simulink model "prac_p3"  (R2024a)
settings: Solver=VariableStepAuto  StartTime=0.0  StopTime=2200  RelTol=1e-3
libraries: simulink x2, slpidlib x1
settings Model: Creator=heman  LastModifiedBy=heman

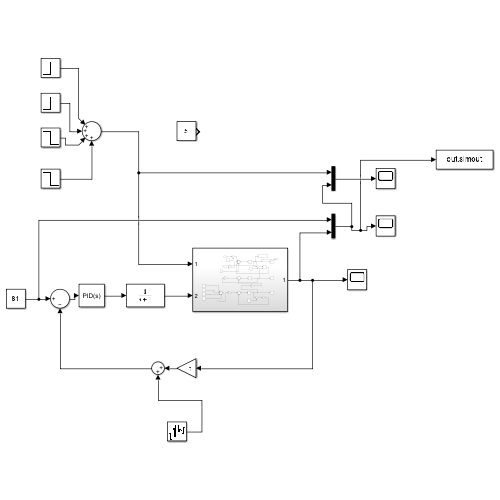
[thumbnail: Simulink's stored preview of the top-level diagram]
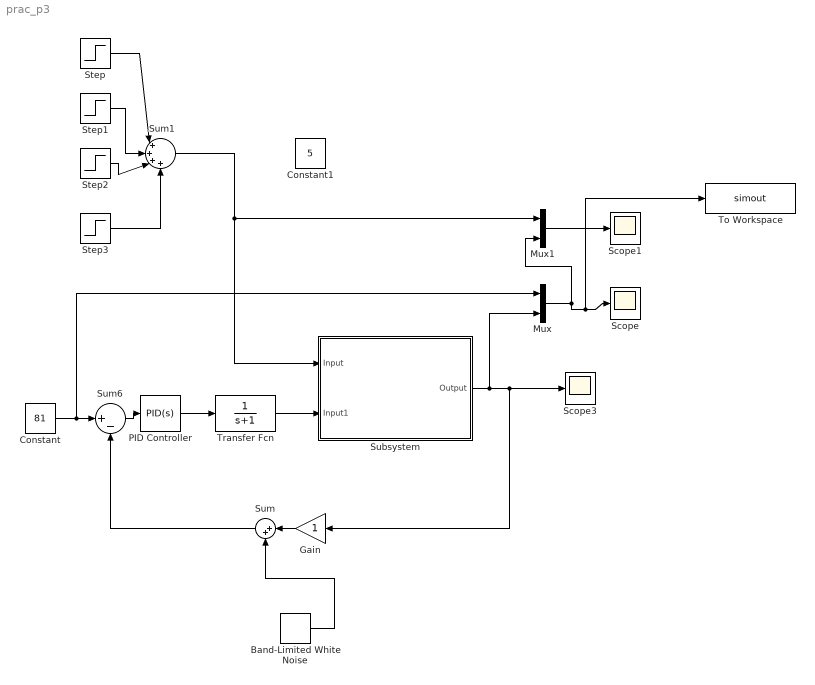
== system prac_p3 ==
  Band-Limited White Noise : simulink/Sources/Band-Limited White Noise  Cov=[0.1]  Ts=0.1  seed=[23341]
  Constant : Constant  Value=81
  Constant1 : Constant  Value=5
  Gain : Gain
  Mux : Mux  Inputs=2
  Mux1 : Mux  Inputs=2
  PID Controller : slpidlib/PID Controller  Controller=PID  Form=Ideal  TimeDomain=Continuous-time  UseExternalTs=off  SampleTime=-1  IntegratorMethod=Forward Euler  FilterMethod=Forward Euler  ControllerParametersSource=internal  P=-0.5078  I=0.01557  UseKiTs=off  D=15.92  UseExternalDerivativeSource=off  N=5.876  UseFilter=on  TunerSelectOption=Transfer Function Based (PID Tuner App)  InitialConditionSource=internal  InitialConditionForIntegrator=0  InitialConditionForFilter=0  DifferentiatorICPrevScaledInput=0  ExternalReset=none  TrackingMode=off  Kt=1  LimitOutput=off  SatLimitsSource=internal  UpperSaturationLimit=inf  LowerSaturationLimit=-inf  LinearizeAsGain=on  AntiWindupMode=none  Kb=1  LimitIntegrator=off  UpperIntegratorSaturationLimit=inf  LowerIntegratorSaturationLimit=-inf  POutMin=[]  POutMax=[]  IOutMin=[]  IOutMax=[]  DOutMin=[]  DOutMax=[]  NOutMin=[]  NOutMax=[]  SumOutMin=[]  SumOutMax=[]  SaturationOutMin=[]  SaturationOutMax=[]  PParamMin=[]  PParamMax=[]  IParamMin=[]  IParamMax=[]  DParamMin=[]  DParamMax=[]  NParamMin=[]  NParamMax=[]  KbParamMin=[]  KbParamMax=[]  KtParamMin=[]  KtParamMax=[]  KbOutMin=[]  KbOutMax=[]  KtOutMin=[]  KtOutMax=[]  IntegratorOutMin=[]  IntegratorOutMax=[]  FilterOutMin=[]  FilterOutMax=[]  SumI1OutMin=[]  SumI1OutMax=[]  SumI2OutMin=[]  SumI2OutMax=[]  SumI3OutMin=[]  SumI3OutMax=[]  SumI4OutMin=[]  SumI4OutMax=[]  SumDOutMin=[]  SumDOutMax=[]  DifferentiatorOutMin=[]  DifferentiatorOutMax=[]  FilterDiffOutCoefMin=[]  FilterDiffOutCoefMax=[]  ReciprocalOutMin=[]  ReciprocalOutMax=[]  SumDenOutMin=[]  SumDenOutMax=[]  SumNumOutMin=[]  SumNumOutMax=[]  DivideOutMin=[]  DivideOutMax=[]  UdiffTsProdOutMin=[]  UdiffTsProdOutMax=[]  NTsProdOutMin=[]  NTsProdOutMax=[]  UintegralTsProdOutMin=[]  UintegralTsProdOutMax=[]  UngainTsProdOutMin=[]  UngainTsProdOutMax=[]  ClampingZeroOutDataTypeStr=Inherit: Inherit via back propagation  ClampingZeroOutMin=[]  ClampingZeroOutMax=[]  FilterDenConstantOutDataTypeStr=Inherit: Inherit via back propagation  FilterDenConstantOutMin=[]  FilterDenConstantOutMax=[]  PCopyOutDataTypeStr=Inherit: Inherit via back propagation  PCopyOutMin=[]  PCopyOutMax=[]  NCopyOutDataTypeStr=Inherit: Inherit via back propagation  NCopyOutMin=[]  NCopyOutMax=[]  IntegratorContinuousStateAttributes=''  IntegratorStateMustResolveToSignalObject=off  IntegratorRTWStateStorageClass=Auto  FilterContinuousStateAttributes=''  FilterStateMustResolveToSignalObject=off  FilterRTWStateStorageClass=Auto  ParallelPVariant=Passthrough  IdealPVariant=InternalParameters  IVariant=InternalParameters  DVariant=InternalParameters  IntegratorVariant=Continuous  SatVariant=Disabled  AWVariant=Passthrough  PCopyVariant=Disabled  TRVariant=Disabled  FdbkBlocksVariant=Forward  IdealPFdbkVariant=Disabled  SatFdbkVariant=Disabled  DerivativeFilterVariant=ContFilter  NVariant=InternalParameters  NCopyVariant=Disabled  FilterICVariant=InternalICsFilter  IntegratorICVariant=InternalICs  ExternalResetVariant=Disabled  TRSumVariant=Passthrough  SumFdbkVariant=Disabled  SumVariant=Sum_PID  TsampFilterVariant=InternalTs  TsampNgainVariant=Passthrough  TsampIntegralVariant=Disabled_SignalSpec  ExternalSaturationOutDataTypeStr=Inherit: Same as second input  DerivativeSourceVariant=ErrorSignal
  Scope : Scope
  Scope1 : Scope
  Scope3 : Scope
  Step : Step  Time=400  Before=5  After=10  SampleTime=0
  Step1 : Step  Time=800  After=5  SampleTime=0
  Step2 : Step  Time=1200  After=-5  SampleTime=0
  Step3 : Step  Time=1600  After=-5  SampleTime=0
  Subsystem : Subsystem
  Sum : Sum  Inputs=|++
  Sum1 : Sum  Inputs=|++++
  Sum6 : Sum  Inputs=|+-
  To Workspace : ToWorkspace  VariableName=simout  SampleTime=-1
  Transfer Fcn : TransferFcn  Denominator=[1 1]
  wires:
  Transfer Fcn/1 -> Subsystem/2(Input1)
  Sum1/1 -> Mux1/1, Subsystem/1(Input)
  PID Controller/1 -> Transfer Fcn/1
  Subsystem/1(Output) -> Scope3/1, Gain/1, Mux/2
  Sum6/1 -> PID Controller/1
  Gain/1 -> Sum/1
  Band-Limited White Noise/1 -> Sum/2
  Sum/1 -> Sum6/2
  Constant/1 -> Mux/1, Sum6/1
  Mux/1 -> Mux1/2, To Workspace/1, Scope/1
  Step2/1 -> Sum1/3
  Step/1 -> Sum1/1
  Step3/1 -> Sum1/4
  Step1/1 -> Sum1/2
  Mux1/1 -> Scope1/1

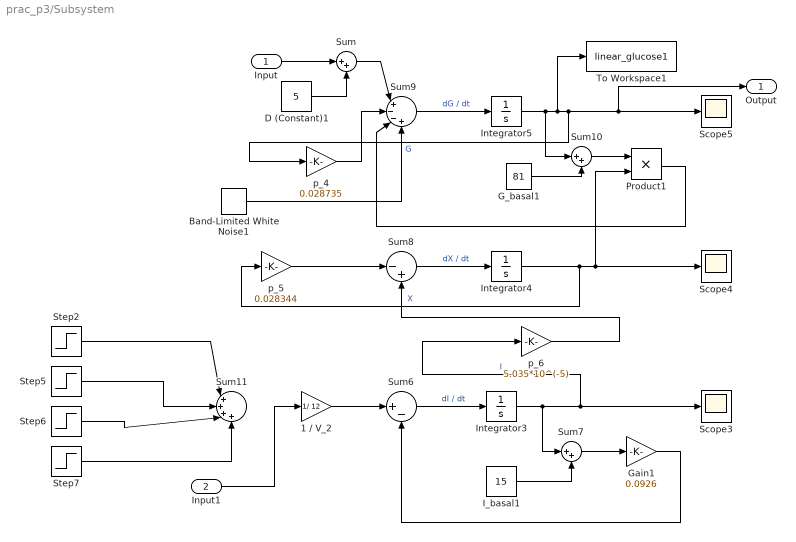
== system prac_p3/Subsystem ==
  Input : Inport
  Input1 : Inport  Port=2
  1 / V_2 : Gain  Gain=1/ 12
  Band-Limited White Noise1 : simulink/Sources/Band-Limited White Noise  Cov=[0.1]  Ts=0.1  seed=[23341]
  D (Constant)1 : Constant  Value=5
  G_basal1 : Constant  Value=81
  Gain1 : Gain  Gain=0.0926
  I_basal1 : Constant  Value=15
  Integrator3 : Integrator
  Integrator4 : Integrator
  Integrator5 : Integrator
  Product1 : Product
  Scope3 : Scope
  Scope4 : Scope
  Scope5 : Scope
  Step2 : Step  Time=500  Before=25  After=27.5  SampleTime=0
  Step5 : Step  Time=1000  After=2.5  SampleTime=0
  Step6 : Step  Time=1500  After=-2.5  SampleTime=0
  Step7 : Step  Time=2000  After=-2.5  SampleTime=0
  Sum : Sum  Inputs=|++
  Sum10 : Sum  Inputs=|++
  Sum11 : Sum  Inputs=|++++
  Sum6 : Sum  Inputs=|+-
  Sum7 : Sum  Inputs=|++
  Sum8 : Sum  Inputs=|-+
  Sum9 : Sum  Inputs=|+--+
  To Workspace1 : ToWorkspace  VariableName=linear_glucose1  SampleTime=-1
  p_4 : Gain  Gain=0.028735
  p_5 : Gain  Gain=0.028344
  p_6 : Gain  Gain=5.035*10^(-5)
  Output : Outport
  wires:
  Integrator4/1 -> p_5/1, Product1/2, Scope4/1  "X"
  Integrator3/1 -> Sum7/1, p_6/1, Scope3/1  "I"
  p_4/1 -> Sum9/2
  Gain1/1 -> Sum6/2
  Sum7/1 -> Gain1/1
  p_6/1 -> Sum8/2
  p_5/1 -> Sum8/1
  Sum9/1 -> Integrator5/1  "dG / dt"
  Step2/1 -> Sum11/1
  Product1/1 -> Sum9/3
  Band-Limited White Noise1/1 -> Sum9/4
  Integrator5/1 -> Sum10/1, To Workspace1/1, p_4/1, Output/1, Scope5/1  "G"
  I_basal1/1 -> Sum7/2
  Sum6/1 -> Integrator3/1  "dI / dt"
  1 / V_2/1 -> Sum6/1
  Sum10/1 -> Product1/1
  D (Constant)1/1 -> Sum/2
  Sum8/1 -> Integrator4/1  "dX / dt"
  Step6/1 -> Sum11/3
  Step5/1 -> Sum11/2
  Step7/1 -> Sum11/4
  G_basal1/1 -> Sum10/2
  Input/1 -> Sum/1
  Sum/1 -> Sum9/1
  Input1/1 -> 1 / V_2/1
